simulink model "angularspeedtospeed"  (R2016b)
settings: Solver=VariableStepAuto  StartTime=0.0  StopTime=10.0  RelTol=1e-3
settings Model: Creator=momen  LastModifiedBy=momen

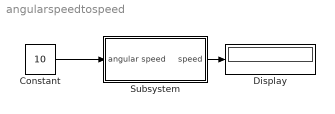
== system angularspeedtospeed ==
  Constant : Constant  Value=10
  Display : Display
  Subsystem : Subsystem
  wires:
  Subsystem/1(" speed") -> Display/1
  Constant/1 -> Subsystem/1(angular speed)

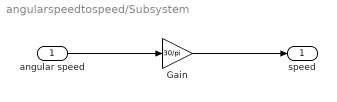
== system angularspeedtospeed/Subsystem ==
  angular speed : Inport
  Gain : Gain  Gain=30/pi
  " speed" : Outport
  wires:
  Gain/1 -> " speed"/1
  angular speed/1 -> Gain/1
